simulink model "AutopilotAssessmentReq1_3"  (R2015b)
settings: Solver=VariableStepAuto  StartTime=0.0  StopTime=10.0  RelTol=1e-3
undefined symbols (not defined in the file or in its folder): msgbox
libraries: simulink x7, sldvlib x4
settings Model: Creator=jdirner  LastModifiedBy=jdirner
settings HardwareCC: ProdWordSize=32

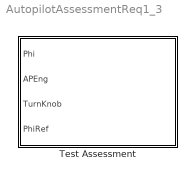
== system AutopilotAssessmentReq1_3 ==
  Test Assessment : Subsystem

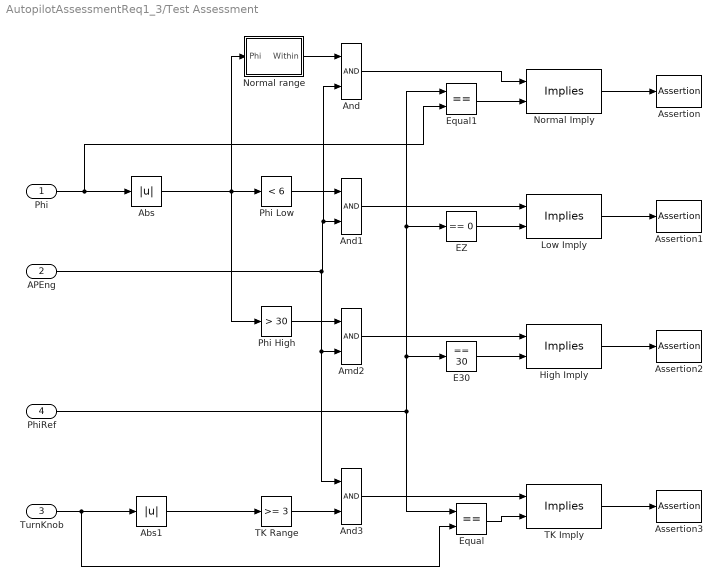
== system AutopilotAssessmentReq1_3/Test Assessment ==
  Phi : Inport
  APEng : Inport  Port=2
  TurnKnob : Inport  Port=3
  PhiRef : Inport  Port=4
  Abs : Abs
  Abs1 : Abs
  Amd2 : Logic  AllPortsSameDT=off  OutDataTypeStr=boolean
  And : Logic  AllPortsSameDT=off  OutDataTypeStr=boolean
  And1 : Logic  AllPortsSameDT=off  OutDataTypeStr=boolean
  And3 : Logic  AllPortsSameDT=off  OutDataTypeStr=boolean
  Assertion : Assertion  AssertionFailFcn=msgbox('PhiRef must equal Phi when Phi within normal range')  StopWhenAssertionFail=off
  Assertion1 : Assertion  AssertionFailFcn=msgbox('PhiRef must equal 0 when Phi < 6 deg')  StopWhenAssertionFail=off
  Assertion2 : Assertion  AssertionFailFcn=msgbox('Phiref must equal 30 when Phi > 30')  StopWhenAssertionFail=off
  Assertion3 : Assertion  AssertionFailFcn=msgbox('PhiRef must equal TurnKnoob setting when TurnKnob >= 3 deg')  StopWhenAssertionFail=off
  E30 : simulink/Logic and Bit Operations/Compare To Constant  relop===  const=30  OutDataTypeStr=boolean
  EZ : simulink/Logic and Bit Operations/Compare To Zero  relop===  OutDataTypeStr=boolean
  Equal : RelationalOperator  Operator===  OutDataTypeStr=boolean
  Equal1 : RelationalOperator  Operator===  OutDataTypeStr=boolean
  High Imply : sldvlib/Verification Utilities/Implies
  Low Imply : sldvlib/Verification Utilities/Implies
  Normal Imply : sldvlib/Verification Utilities/Implies
  Normal range : Subsystem
  Phi High : simulink/Logic and Bit Operations/Compare To Constant  relop=>  const=30  OutDataTypeStr=boolean
  Phi Low : simulink/Logic and Bit Operations/Compare To Constant  relop=<  const=6  OutDataTypeStr=boolean
  TK Imply : sldvlib/Verification Utilities/Implies
  TK Range : simulink/Logic and Bit Operations/Compare To Constant  relop=>=  const=3  OutDataTypeStr=boolean
  wires:
  APEng/1 -> And3/1, Amd2/2, And/2, And1/2
  Phi/1 -> Equal1/2, Abs/1
  Phi Low/1 -> And1/1
  EZ/1 -> Low Imply/2
  PhiRef/1 -> E30/1, Equal1/1, EZ/1, Equal/1
  And1/1 -> Low Imply/1
  Phi High/1 -> Amd2/1
  E30/1 -> High Imply/2
  Amd2/1 -> High Imply/1
  Abs/1 -> Normal range/1(Phi), Phi High/1, Phi Low/1
  TurnKnob/1 -> Equal/2, Abs1/1
  Abs1/1 -> TK Range/1
  TK Range/1 -> And3/2
  And3/1 -> TK Imply/1
  Equal/1 -> TK Imply/2
  Normal range/1(Within) -> And/1
  Equal1/1 -> Normal Imply/2
  And/1 -> Normal Imply/1
  Low Imply/1 -> Assertion1/1
  High Imply/1 -> Assertion2/1
  TK Imply/1 -> Assertion3/1
  Normal Imply/1 -> Assertion/1

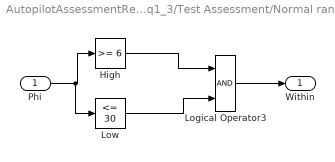
== system AutopilotAssessmentReq1_3/Test Assessment/Normal range ==
  Phi : Inport
  High : simulink/Logic and Bit Operations/Compare To Constant  relop=>=  const=6  OutDataTypeStr=boolean
  Logical Operator3 : Logic  AllPortsSameDT=off  OutDataTypeStr=boolean
  Low : simulink/Logic and Bit Operations/Compare To Constant  relop=<=  const=30  OutDataTypeStr=boolean
  Within : Outport
  wires:
  Low/1 -> Logical Operator3/2
  Phi/1 -> Low/1, High/1
  High/1 -> Logical Operator3/1
  Logical Operator3/1 -> Within/1
